simulink model "fsm_12B_with_contracts_PP"  (R2017b)
settings: Solver=FixedStepDiscrete  StartTime=0.0  StopTime=10  FixedStep=0.200000  RelTol=1e-3  EnableMultiTasking=on
model workspace (MAT data in the model file):
  MCOS : class17 (value not decoded)
  already_pp = 1
  compositionalMap : struct (value not decoded)
  MCOS : class17 (value not decoded)
  MCOS : class17 (value not decoded)
  verificationResults : struct (value not decoded)
undefined symbols (not defined in the file): contractAfterSimulation, contractBeforeSimulation, ContractBlock, ContractGuaranteeBlock, ContractValidatorBlock, saveValidatorParameters
(part 2 of 2)

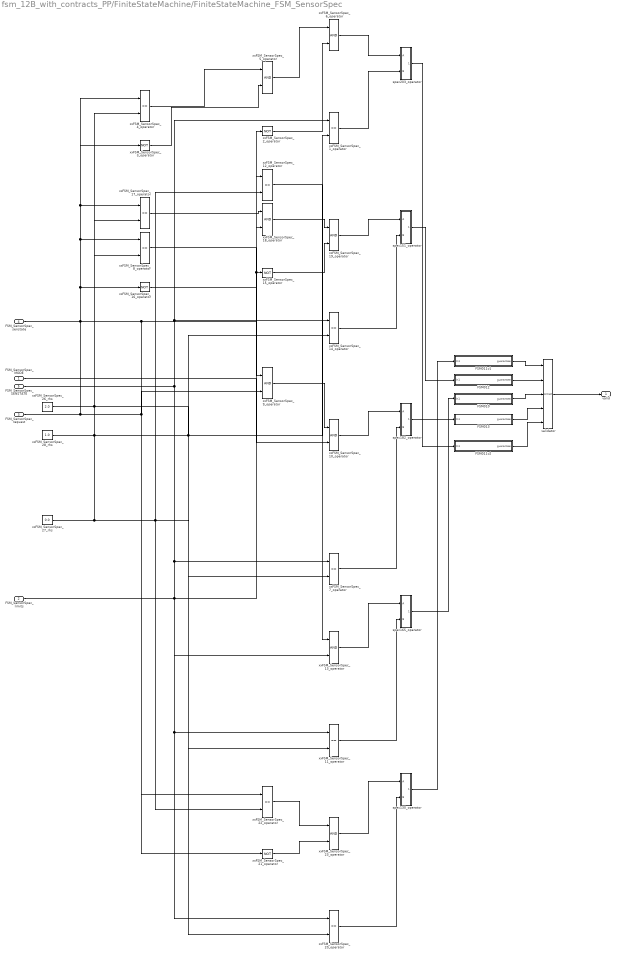
== system fsm_12B_with_contracts_PP/FiniteStateMachine/FiniteStateMachine_FSM_SensorSpec ==
  FSM_SensorSpec_MODE : Inport  OutDataTypeStr=boolean
  FSM_SensorSpec_limits : Inport  Port=2  OutDataTypeStr=boolean
  FSM_SensorSpec_request : Inport  Port=3  OutDataTypeStr=boolean
  FSM_SensorSpec_senstate : Inport  Port=4  OutDataTypeStr=double
  FSM_SensorSpec_SENSTATE : Inport  Port=5  OutDataTypeStr=double
  FSM010 : Subsystem  TreatAsAtomicUnit=on  mask(ContractGuaranteeBlock){ContractBlockType=ContractGuaranteeBlock}
      mask init:
      | set_param(gcb, 'LinkStatus', 'none');
      mask DialogControl DescTextVar Prompt: Guarantee block
  FSM011v1 : Subsystem  TreatAsAtomicUnit=on  mask(ContractGuaranteeBlock){ContractBlockType=ContractGuaranteeBlock}
      mask init:
      | set_param(gcb, 'LinkStatus', 'none');
      mask DialogControl DescTextVar Prompt: Guarantee block
      mask DialogControl Display_counter_example_as_signals Prompt: Display counter example as signals
      mask DialogControl Display_counter_example_as_signals Callback: displayCexSignals(1, 1);
      mask DialogControl Display_counter_example_as_tables Prompt: Display counter example as tables
      mask DialogControl Display_counter_example_as_tables Callback: displayCexTables(1, 1);
      mask DialogControl Display_counter_example_as_HTML_tables Prompt: Display counter example as HTML tables
      mask DialogControl Display_counter_example_as_HTML_tables Callback: displayCexHtmlTables(1, 1);
      mask DialogControl Generate_an_outer_model_for_the_counter_example Prompt: Generate an outer model for the counter example
      mask DialogControl Generate_an_outer_model_for_the_counter_example Callback: generateModelWithSignalBuilders(1, 1, 2);
      mask DialogControl Generate_an_inner_model_for_the_counter_example Prompt: Generate an inner model for the counter example
      mask DialogControl Generate_an_inner_model_for_the_counter_example Callback: generateModelWithSignalBuilders(1, 1, 1);
  FSM011v2 : Subsystem  TreatAsAtomicUnit=on  mask(ContractGuaranteeBlock){ContractBlockType=ContractGuaranteeBlock}
      mask init:
      | set_param(gcb, 'LinkStatus', 'none');
      mask DialogControl DescTextVar Prompt: Guarantee block
  FSM012 : Subsystem  TreatAsAtomicUnit=on  mask(ContractGuaranteeBlock){ContractBlockType=ContractGuaranteeBlock}
      mask init:
      | set_param(gcb, 'LinkStatus', 'none');
      mask DialogControl DescTextVar Prompt: Guarantee block
  FSM013 : Subsystem  TreatAsAtomicUnit=on  mask(ContractGuaranteeBlock){ContractBlockType=ContractGuaranteeBlock}
      mask init:
      | set_param(gcb, 'LinkStatus', 'none');
      mask DialogControl DescTextVar Prompt: Guarantee block
  spec130_operator : Subsystem  TreatAsAtomicUnit=on
  spec151_operator : Subsystem  TreatAsAtomicUnit=on
  spec165_operator : Subsystem  TreatAsAtomicUnit=on
  spec182_operator : Subsystem  TreatAsAtomicUnit=on
  spec203_operator : Subsystem  TreatAsAtomicUnit=on
  validator : M-S-Function  LoadFcn=saveValidatorParameters(gcb);  InitFcn=contractBeforeSimulation();  StopFcn=contractAfterSimulation();  FunctionName=contract  mask(ContractValidatorBlock){assumePorts=0, guaranteePorts=5, modePorts=0, ContractBlockType=ContractValidatorBlock, createInportsCheckbox=off}
      mask prompts: assumePorts "Assume ports     :"; guaranteePorts "Guarantee ports :"; modePorts "Mode ports        :"; createInportsCheckbox "Create inports and connect them automatically"
      mask init:
      | set_param(gcb,'LinkStatus','none');
      | contract_callback('inputs_callback',gcb);
      mask DialogControl DescTextVar Prompt: The validator block implements the following logic: <br> <br> <b>Sofar</b>(assume<sub>1</sub> <b>&#8743;</b> assume<sub>2</sub> <b>&#8743;</b> ... assume<sub>k</sub>) <b>&rarr;</b> (guarantee<sub>1</sub> <b>&#8743;</b> guarantee<sub>2</sub> <b>&#8743;</b> ... guarantee<sub>m</sub> <b>&#8743;</b>  mode<sub>1</sub> <b>&#8743;</b> mode<sub>2</sub> <b>&#8743;</b> ... <b>&#8743;</b> mode<sub>n</sub> )<br> where mode<sub>i</sub> = require<sub>i</sub> <b>&rarr;</b> ensure<sub>i</sub>
      mask Display:
      | color('black');
      | port_label('input',1,'guarantee');
      | port_label('input',2,'guarantee');
      | port_label('input',3,'guarantee');
      | port_label('input',4,'guarantee');
      | port_label('input',5,'guarantee');
      | port_label('output',1,'valid');
  xxFSM_SensorSpec_10_operator : Logic  AllPortsSameDT=off  OutDataTypeStr=boolean
  xxFSM_SensorSpec_11_operator : RelationalOperator  Operator===  OutDataTypeStr=boolean  RndMeth=Simplest
  xxFSM_SensorSpec_12_operator : RelationalOperator  Operator===  OutDataTypeStr=boolean  RndMeth=Simplest
  xxFSM_SensorSpec_13_operator : Logic  AllPortsSameDT=off  OutDataTypeStr=boolean
  xxFSM_SensorSpec_14_operator : RelationalOperator  Operator===  OutDataTypeStr=boolean  RndMeth=Simplest
  xxFSM_SensorSpec_15_operator : Logic  Operator=NOT  AllPortsSameDT=off  OutDataTypeStr=boolean
  xxFSM_SensorSpec_16_operator : Logic  Operator=NOT  AllPortsSameDT=off  OutDataTypeStr=boolean
  xxFSM_SensorSpec_17_operator : RelationalOperator  Operator===  OutDataTypeStr=boolean  RndMeth=Simplest
  xxFSM_SensorSpec_18_operator : Logic  AllPortsSameDT=off  OutDataTypeStr=boolean
  xxFSM_SensorSpec_19_operator : Logic  AllPortsSameDT=off  OutDataTypeStr=boolean
  xxFSM_SensorSpec_1_operator : RelationalOperator  Operator===  OutDataTypeStr=boolean  RndMeth=Simplest
  xxFSM_SensorSpec_20_operator : RelationalOperator  Operator===  OutDataTypeStr=boolean  RndMeth=Simplest
  xxFSM_SensorSpec_21_operator : Logic  Operator=NOT  AllPortsSameDT=off  OutDataTypeStr=boolean
  xxFSM_SensorSpec_22_operator : RelationalOperator  Operator===  OutDataTypeStr=boolean  RndMeth=Simplest
  xxFSM_SensorSpec_23_operator : Logic  AllPortsSameDT=off  OutDataTypeStr=boolean
  xxFSM_SensorSpec_26_rhs : Constant  Value=2.0  OutDataTypeStr=double
  xxFSM_SensorSpec_27_rhs : Constant  Value=0.0  OutDataTypeStr=double
  xxFSM_SensorSpec_28_rhs : Constant  Value=1.0  OutDataTypeStr=double
  xxFSM_SensorSpec_2_operator : Logic  Operator=NOT  AllPortsSameDT=off  OutDataTypeStr=boolean
  xxFSM_SensorSpec_3_operator : Logic  Operator=NOT  AllPortsSameDT=off  OutDataTypeStr=boolean
  xxFSM_SensorSpec_4_operator : RelationalOperator  Operator===  OutDataTypeStr=boolean  RndMeth=Simplest
  xxFSM_SensorSpec_5_operator : Logic  AllPortsSameDT=off  OutDataTypeStr=boolean
  xxFSM_SensorSpec_6_operator : Logic  AllPortsSameDT=off  OutDataTypeStr=boolean
  xxFSM_SensorSpec_7_operator : RelationalOperator  Operator===  OutDataTypeStr=boolean  RndMeth=Simplest
  xxFSM_SensorSpec_8_operator : RelationalOperator  Operator===  OutDataTypeStr=boolean  RndMeth=Simplest
  xxFSM_SensorSpec_9_operator : Logic  AllPortsSameDT=off  OutDataTypeStr=boolean
  valid : Outport
  wires:
  validator/1 -> valid/1
  xxFSM_SensorSpec_8_operator/1 -> xxFSM_SensorSpec_9_operator/1
  xxFSM_SensorSpec_2_operator/1 -> xxFSM_SensorSpec_6_operator/2
  xxFSM_SensorSpec_5_operator/1 -> xxFSM_SensorSpec_6_operator/1
  xxFSM_SensorSpec_3_operator/1 -> xxFSM_SensorSpec_5_operator/2
  xxFSM_SensorSpec_4_operator/1 -> xxFSM_SensorSpec_5_operator/1
  xxFSM_SensorSpec_21_operator/1 -> xxFSM_SensorSpec_23_operator/2
  xxFSM_SensorSpec_22_operator/1 -> xxFSM_SensorSpec_23_operator/1
  xxFSM_SensorSpec_15_operator/1 -> xxFSM_SensorSpec_19_operator/2
  xxFSM_SensorSpec_18_operator/1 -> xxFSM_SensorSpec_19_operator/1
  xxFSM_SensorSpec_16_operator/1 -> xxFSM_SensorSpec_18_operator/2
  xxFSM_SensorSpec_17_operator/1 -> xxFSM_SensorSpec_18_operator/1
  xxFSM_SensorSpec_12_operator/1 -> xxFSM_SensorSpec_13_operator/1
  FSM_SensorSpec_MODE/1 -> xxFSM_SensorSpec_10_operator/2
  xxFSM_SensorSpec_9_operator/1 -> xxFSM_SensorSpec_10_operator/1
  FSM011v2/1(guarantee) -> validator/5
  FSM013/1(guarantee) -> validator/4
  FSM010/1(guarantee) -> validator/3
  FSM012/1(guarantee) -> validator/2
  FSM011v1/1(guarantee) -> validator/1
  xxFSM_SensorSpec_1_operator/1 -> spec203_operator/2(B)
  xxFSM_SensorSpec_6_operator/1 -> spec203_operator/1(A)
  xxFSM_SensorSpec_7_operator/1 -> spec182_operator/2(B)
  xxFSM_SensorSpec_10_operator/1 -> spec182_operator/1(A)
  xxFSM_SensorSpec_11_operator/1 -> spec165_operator/2(B)
  xxFSM_SensorSpec_13_operator/1 -> spec165_operator/1(A)
  xxFSM_SensorSpec_14_operator/1 -> spec151_operator/2(B)
  xxFSM_SensorSpec_19_operator/1 -> spec151_operator/1(A)
  xxFSM_SensorSpec_20_operator/1 -> spec130_operator/2(B)
  xxFSM_SensorSpec_23_operator/1 -> spec130_operator/1(A)
  spec203_operator/1(A_equal__equal__gt_B) -> FSM011v2/1(In1)
  spec182_operator/1(A_equal__equal__gt_B) -> FSM013/1(In1)
  spec165_operator/1(A_equal__equal__gt_B) -> FSM010/1(In1)
  spec151_operator/1(A_equal__equal__gt_B) -> FSM012/1(In1)
  spec130_operator/1(A_equal__equal__gt_B) -> FSM011v1/1(In1)
  xxFSM_SensorSpec_28_rhs/1 -> xxFSM_SensorSpec_20_operator/2, xxFSM_SensorSpec_1_operator/2, xxFSM_SensorSpec_14_operator/2, xxFSM_SensorSpec_8_operator/2
  FSM_SensorSpec_request/1 -> xxFSM_SensorSpec_9_operator/2, xxFSM_SensorSpec_21_operator/1, xxFSM_SensorSpec_3_operator/1, xxFSM_SensorSpec_16_operator/1
  xxFSM_SensorSpec_26_rhs/1 -> xxFSM_SensorSpec_17_operator/2, xxFSM_SensorSpec_11_operator/2
  FSM_SensorSpec_SENSTATE/1 -> xxFSM_SensorSpec_20_operator/1, xxFSM_SensorSpec_11_operator/1, xxFSM_SensorSpec_7_operator/1, xxFSM_SensorSpec_1_operator/1, xxFSM_SensorSpec_14_operator/1
  FSM_SensorSpec_limits/1 -> xxFSM_SensorSpec_2_operator/1, xxFSM_SensorSpec_15_operator/1, xxFSM_SensorSpec_13_operator/2
  xxFSM_SensorSpec_27_rhs/1 -> xxFSM_SensorSpec_7_operator/2, xxFSM_SensorSpec_22_operator/2, xxFSM_SensorSpec_12_operator/2, xxFSM_SensorSpec_4_operator/2
  FSM_SensorSpec_senstate/1 -> xxFSM_SensorSpec_22_operator/1, xxFSM_SensorSpec_12_operator/1, xxFSM_SensorSpec_4_operator/1, xxFSM_SensorSpec_17_operator/1, xxFSM_SensorSpec_8_operator/1

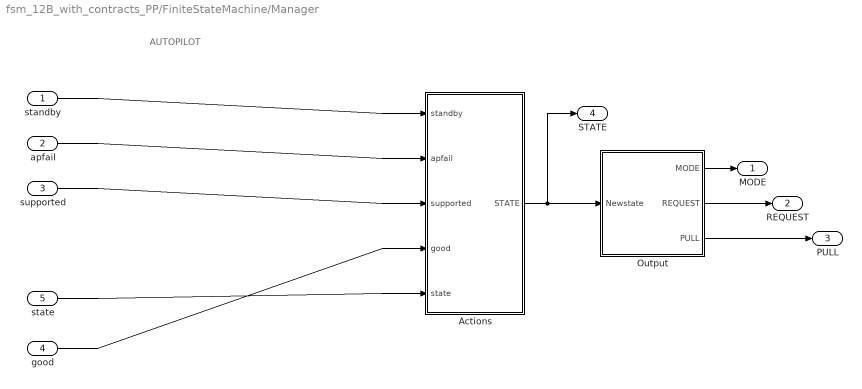
== system fsm_12B_with_contracts_PP/FiniteStateMachine/Manager ==
  note: AUTOPILOT
  standby : Inport
  apfail : Inport  Port=2
  supported : Inport  Port=3
  good : Inport  Port=4
  state : Inport  Port=5
  Actions : Subsystem  TreatAsAtomicUnit=on
  Output : Subsystem  TreatAsAtomicUnit=on
  MODE : Outport  VectorParamsAs1DForOutWhenUnconnected=off
  REQUEST : Outport  Port=2  VectorParamsAs1DForOutWhenUnconnected=off
  PULL : Outport  Port=3  VectorParamsAs1DForOutWhenUnconnected=off
  STATE : Outport  Port=4  VectorParamsAs1DForOutWhenUnconnected=off
  wires:
  Actions/1(STATE) -> STATE/1, Output/1(Newstate)
  apfail/1 -> Actions/2(apfail)
  state/1 -> Actions/5(state)
  supported/1 -> Actions/3(supported)
  good/1 -> Actions/4(good)
  standby/1 -> Actions/1(standby)
  Output/1(MODE) -> MODE/1
  Output/2(REQUEST) -> REQUEST/1
  Output/3(PULL) -> PULL/1

== system fsm_12B_with_contracts_PP/FiniteStateMachine/Sen ==
  note: SENSOR
  mode : Inport
  request : Inport  Port=2
  limits : Inport  Port=3
  senstate : Inport  Port=4
  Actions : Subsystem  TreatAsAtomicUnit=on
  Output : Subsystem  TreatAsAtomicUnit=on
  good : Outport  VectorParamsAs1DForOutWhenUnconnected=off
  SENSTATE : Outport  Port=2  VectorParamsAs1DForOutWhenUnconnected=off
  wires:
  Output/1(Good) -> good/1
  request/1 -> Actions/2(request)
  mode/1 -> Actions/1(mode)
  Actions/1(SENSTATE) -> Output/1(Newstate), SENSTATE/1
  senstate/1 -> Actions/4(senstate)
  limits/1 -> Actions/3(limits)

== system fsm_12B_with_contracts_PP/fsm_12B_FSMSpec/FSM001v1 ==
  In1 : Inport
  guarantee : Outport  OutDataTypeStr=boolean
  wires:
  In1/1 -> guarantee/1

== system fsm_12B_with_contracts_PP/fsm_12B_FSMSpec/FSM001v2 ==
  In1 : Inport
  guarantee : Outport  OutDataTypeStr=boolean
  wires:
  In1/1 -> guarantee/1

== system fsm_12B_with_contracts_PP/fsm_12B_FSMSpec/FSM001v3 ==
  In1 : Inport
  guarantee : Outport  OutDataTypeStr=boolean
  wires:
  In1/1 -> guarantee/1

== system fsm_12B_with_contracts_PP/fsm_12B_FSMSpec/HT_call ==
  HT_L : Inport
  HT_R : Inport  Port=2
  HT_X : Inport  Port=3  OutDataTypeStr=boolean
  OT_call : Subsystem  TreatAsAtomicUnit=on
  Y_operator : Logic  Operator=NOT  AllPortsSameDT=off  OutDataTypeStr=boolean
  xxHT_1_operator : Logic  Operator=NOT  AllPortsSameDT=off  OutDataTypeStr=boolean
  HT_Y : Outport
  wires:
  Y_operator/1 -> HT_Y/1
  HT_X/1 -> xxHT_1_operator/1
  OT_call/1(OT_Y) -> Y_operator/1
  xxHT_1_operator/1 -> OT_call/3(OT_X)
  HT_R/1 -> OT_call/2(OT_R)
  HT_L/1 -> OT_call/1(OT_L)

== system fsm_12B_with_contracts_PP/fsm_12B_FSMSpec/HT_call1 ==
  HT_L : Inport
  HT_R : Inport  Port=2
  HT_X : Inport  Port=3  OutDataTypeStr=boolean
  OT_call : Subsystem  TreatAsAtomicUnit=on
  Y_operator : Logic  Operator=NOT  AllPortsSameDT=off  OutDataTypeStr=boolean
  xxHT_1_operator : Logic  Operator=NOT  AllPortsSameDT=off  OutDataTypeStr=boolean
  HT_Y : Outport
  wires:
  Y_operator/1 -> HT_Y/1
  HT_X/1 -> xxHT_1_operator/1
  OT_call/1(OT_Y) -> Y_operator/1
  xxHT_1_operator/1 -> OT_call/3(OT_X)
  HT_R/1 -> OT_call/2(OT_R)
  HT_L/1 -> OT_call/1(OT_L)

== system fsm_12B_with_contracts_PP/fsm_12B_FSMSpec/spec166_operator ==
  A : Inport
  B : Inport  Port=2
  Logical_newline_Operator : Logic  Operator=OR  AllPortsSameDT=off  OutDataTypeStr=boolean
  Logical_newline_Operator1 : Logic  Operator=NOT  AllPortsSameDT=off  OutDataTypeStr=boolean
  A_equal__equal__gt_B : Outport  VectorParamsAs1DForOutWhenUnconnected=off
  wires:
  B/1 -> Logical_newline_Operator/2
  A/1 -> Logical_newline_Operator1/1
  Logical_newline_Operator/1 -> A_equal__equal__gt_B/1
  Logical_newline_Operator1/1 -> Logical_newline_Operator/1

== system fsm_12B_with_contracts_PP/fsm_12B_FSMSpec/spec194_operator ==
  A : Inport
  B : Inport  Port=2
  Logical_newline_Operator : Logic  Operator=OR  AllPortsSameDT=off  OutDataTypeStr=boolean
  Logical_newline_Operator1 : Logic  Operator=NOT  AllPortsSameDT=off  OutDataTypeStr=boolean
  A_equal__equal__gt_B : Outport  VectorParamsAs1DForOutWhenUnconnected=off
  wires:
  B/1 -> Logical_newline_Operator/2
  A/1 -> Logical_newline_Operator1/1
  Logical_newline_Operator/1 -> A_equal__equal__gt_B/1
  Logical_newline_Operator1/1 -> Logical_newline_Operator/1

== system fsm_12B_with_contracts_PP/fsm_12B_FSMSpec/spec222_operator ==
  A : Inport
  B : Inport  Port=2
  Logical_newline_Operator : Logic  Operator=OR  AllPortsSameDT=off  OutDataTypeStr=boolean
  Logical_newline_Operator1 : Logic  Operator=NOT  AllPortsSameDT=off  OutDataTypeStr=boolean
  A_equal__equal__gt_B : Outport  VectorParamsAs1DForOutWhenUnconnected=off
  wires:
  B/1 -> Logical_newline_Operator/2
  A/1 -> Logical_newline_Operator1/1
  Logical_newline_Operator/1 -> A_equal__equal__gt_B/1
  Logical_newline_Operator1/1 -> Logical_newline_Operator/1

== system fsm_12B_with_contracts_PP/FiniteStateMachine/FiniteStateMachine_FSM_AutopilotSpec1/FSM002 ==
  In1 : Inport
  guarantee : Outport  OutDataTypeStr=boolean
  wires:
  In1/1 -> guarantee/1

== system fsm_12B_with_contracts_PP/FiniteStateMachine/FiniteStateMachine_FSM_AutopilotSpec1/FSM003 ==
  In1 : Inport
  guarantee : Outport  OutDataTypeStr=boolean
  wires:
  In1/1 -> guarantee/1

== system fsm_12B_with_contracts_PP/FiniteStateMachine/FiniteStateMachine_FSM_AutopilotSpec1/FSM003v2 ==
  In1 : Inport
  guarantee : Outport  OutDataTypeStr=boolean
  wires:
  In1/1 -> guarantee/1

== system fsm_12B_with_contracts_PP/FiniteStateMachine/FiniteStateMachine_FSM_AutopilotSpec1/FSM004 ==
  In1 : Inport
  guarantee : Outport  OutDataTypeStr=boolean
  wires:
  In1/1 -> guarantee/1

== system fsm_12B_with_contracts_PP/FiniteStateMachine/FiniteStateMachine_FSM_AutopilotSpec1/FSM004v2 ==
  In1 : Inport
  guarantee : Outport  OutDataTypeStr=boolean
  wires:
  In1/1 -> guarantee/1

== system fsm_12B_with_contracts_PP/FiniteStateMachine/FiniteStateMachine_FSM_AutopilotSpec1/FSM005 ==
  In1 : Inport
  guarantee : Outport  OutDataTypeStr=boolean
  wires:
  In1/1 -> guarantee/1

== system fsm_12B_with_contracts_PP/FiniteStateMachine/FiniteStateMachine_FSM_AutopilotSpec1/FSM006 ==
  In1 : Inport
  guarantee : Outport  OutDataTypeStr=boolean
  wires:
  In1/1 -> guarantee/1

== system fsm_12B_with_contracts_PP/FiniteStateMachine/FiniteStateMachine_FSM_AutopilotSpec1/FSM007 ==
  In1 : Inport
  guarantee : Outport  OutDataTypeStr=boolean
  wires:
  In1/1 -> guarantee/1

== system fsm_12B_with_contracts_PP/FiniteStateMachine/FiniteStateMachine_FSM_AutopilotSpec1/FSM007v2 ==
  In1 : Inport
  guarantee : Outport  OutDataTypeStr=boolean
  wires:
  In1/1 -> guarantee/1

== system fsm_12B_with_contracts_PP/FiniteStateMachine/FiniteStateMachine_FSM_AutopilotSpec1/FSM008v1 ==
  In1 : Inport
  guarantee : Outport  OutDataTypeStr=boolean
  wires:
  In1/1 -> guarantee/1

== system fsm_12B_with_contracts_PP/FiniteStateMachine/FiniteStateMachine_FSM_AutopilotSpec1/FSM008v2 ==
  In1 : Inport
  guarantee : Outport  OutDataTypeStr=boolean
  wires:
  In1/1 -> guarantee/1

== system fsm_12B_with_contracts_PP/FiniteStateMachine/FiniteStateMachine_FSM_AutopilotSpec1/FSM009 ==
  In1 : Inport
  guarantee : Outport  OutDataTypeStr=boolean
  wires:
  In1/1 -> guarantee/1

== system fsm_12B_with_contracts_PP/FiniteStateMachine/FiniteStateMachine_FSM_AutopilotSpec1/spec129_operator ==
  A : Inport
  B : Inport  Port=2
  Logical_newline_Operator : Logic  Operator=OR  AllPortsSameDT=off  OutDataTypeStr=boolean
  Logical_newline_Operator1 : Logic  Operator=NOT  AllPortsSameDT=off  OutDataTypeStr=boolean
  A_equal__equal__gt_B : Outport  VectorParamsAs1DForOutWhenUnconnected=off
  wires:
  Logical_newline_Operator1/1 -> Logical_newline_Operator/1
  Logical_newline_Operator/1 -> A_equal__equal__gt_B/1
  A/1 -> Logical_newline_Operator1/1
  B/1 -> Logical_newline_Operator/2

== system fsm_12B_with_contracts_PP/FiniteStateMachine/FiniteStateMachine_FSM_AutopilotSpec1/spec143_operator ==
  A : Inport
  B : Inport  Port=2
  Logical_newline_Operator : Logic  Operator=OR  AllPortsSameDT=off  OutDataTypeStr=boolean
  Logical_newline_Operator1 : Logic  Operator=NOT  AllPortsSameDT=off  OutDataTypeStr=boolean
  A_equal__equal__gt_B : Outport  VectorParamsAs1DForOutWhenUnconnected=off
  wires:
  Logical_newline_Operator1/1 -> Logical_newline_Operator/1
  Logical_newline_Operator/1 -> A_equal__equal__gt_B/1
  A/1 -> Logical_newline_Operator1/1
  B/1 -> Logical_newline_Operator/2

== system fsm_12B_with_contracts_PP/FiniteStateMachine/FiniteStateMachine_FSM_AutopilotSpec1/spec160_operator ==
  A : Inport
  B : Inport  Port=2
  Logical_newline_Operator : Logic  Operator=OR  AllPortsSameDT=off  OutDataTypeStr=boolean
  Logical_newline_Operator1 : Logic  Operator=NOT  AllPortsSameDT=off  OutDataTypeStr=boolean
  A_equal__equal__gt_B : Outport  VectorParamsAs1DForOutWhenUnconnected=off
  wires:
  Logical_newline_Operator1/1 -> Logical_newline_Operator/1
  Logical_newline_Operator/1 -> A_equal__equal__gt_B/1
  A/1 -> Logical_newline_Operator1/1
  B/1 -> Logical_newline_Operator/2

== system fsm_12B_with_contracts_PP/FiniteStateMachine/FiniteStateMachine_FSM_AutopilotSpec1/spec182_operator ==
  A : Inport
  B : Inport  Port=2
  Logical_newline_Operator : Logic  Operator=OR  AllPortsSameDT=off  OutDataTypeStr=boolean
  Logical_newline_Operator1 : Logic  Operator=NOT  AllPortsSameDT=off  OutDataTypeStr=boolean
  A_equal__equal__gt_B : Outport  VectorParamsAs1DForOutWhenUnconnected=off
  wires:
  Logical_newline_Operator1/1 -> Logical_newline_Operator/1
  Logical_newline_Operator/1 -> A_equal__equal__gt_B/1
  A/1 -> Logical_newline_Operator1/1
  B/1 -> Logical_newline_Operator/2

== system fsm_12B_with_contracts_PP/FiniteStateMachine/FiniteStateMachine_FSM_AutopilotSpec1/spec198_operator ==
  A : Inport
  B : Inport  Port=2
  Logical_newline_Operator : Logic  Operator=OR  AllPortsSameDT=off  OutDataTypeStr=boolean
  Logical_newline_Operator1 : Logic  Operator=NOT  AllPortsSameDT=off  OutDataTypeStr=boolean
  A_equal__equal__gt_B : Outport  VectorParamsAs1DForOutWhenUnconnected=off
  wires:
  Logical_newline_Operator1/1 -> Logical_newline_Operator/1
  Logical_newline_Operator/1 -> A_equal__equal__gt_B/1
  A/1 -> Logical_newline_Operator1/1
  B/1 -> Logical_newline_Operator/2

== system fsm_12B_with_contracts_PP/FiniteStateMachine/FiniteStateMachine_FSM_AutopilotSpec1/spec212_operator ==
  A : Inport
  B : Inport  Port=2
  Logical_newline_Operator : Logic  Operator=OR  AllPortsSameDT=off  OutDataTypeStr=boolean
  Logical_newline_Operator1 : Logic  Operator=NOT  AllPortsSameDT=off  OutDataTypeStr=boolean
  A_equal__equal__gt_B : Outport  VectorParamsAs1DForOutWhenUnconnected=off
  wires:
  Logical_newline_Operator1/1 -> Logical_newline_Operator/1
  Logical_newline_Operator/1 -> A_equal__equal__gt_B/1
  A/1 -> Logical_newline_Operator1/1
  B/1 -> Logical_newline_Operator/2

== system fsm_12B_with_contracts_PP/FiniteStateMachine/FiniteStateMachine_FSM_AutopilotSpec1/spec233_operator ==
  A : Inport
  B : Inport  Port=2
  Logical_newline_Operator : Logic  Operator=OR  AllPortsSameDT=off  OutDataTypeStr=boolean
  Logical_newline_Operator1 : Logic  Operator=NOT  AllPortsSameDT=off  OutDataTypeStr=boolean
  A_equal__equal__gt_B : Outport  VectorParamsAs1DForOutWhenUnconnected=off
  wires:
  Logical_newline_Operator1/1 -> Logical_newline_Operator/1
  Logical_newline_Operator/1 -> A_equal__equal__gt_B/1
  A/1 -> Logical_newline_Operator1/1
  B/1 -> Logical_newline_Operator/2

== system fsm_12B_with_contracts_PP/FiniteStateMachine/FiniteStateMachine_FSM_AutopilotSpec1/spec254_operator ==
  A : Inport
  B : Inport  Port=2
  Logical_newline_Operator : Logic  Operator=OR  AllPortsSameDT=off  OutDataTypeStr=boolean
  Logical_newline_Operator1 : Logic  Operator=NOT  AllPortsSameDT=off  OutDataTypeStr=boolean
  A_equal__equal__gt_B : Outport  VectorParamsAs1DForOutWhenUnconnected=off
  wires:
  Logical_newline_Operator1/1 -> Logical_newline_Operator/1
  Logical_newline_Operator/1 -> A_equal__equal__gt_B/1
  A/1 -> Logical_newline_Operator1/1
  B/1 -> Logical_newline_Operator/2

== system fsm_12B_with_contracts_PP/FiniteStateMachine/FiniteStateMachine_FSM_AutopilotSpec1/spec271_operator ==
  A : Inport
  B : Inport  Port=2
  Logical_newline_Operator : Logic  Operator=OR  AllPortsSameDT=off  OutDataTypeStr=boolean
  Logical_newline_Operator1 : Logic  Operator=NOT  AllPortsSameDT=off  OutDataTypeStr=boolean
  A_equal__equal__gt_B : Outport  VectorParamsAs1DForOutWhenUnconnected=off
  wires:
  Logical_newline_Operator1/1 -> Logical_newline_Operator/1
  Logical_newline_Operator/1 -> A_equal__equal__gt_B/1
  A/1 -> Logical_newline_Operator1/1
  B/1 -> Logical_newline_Operator/2

== system fsm_12B_with_contracts_PP/FiniteStateMachine/FiniteStateMachine_FSM_AutopilotSpec1/spec287_operator ==
  A : Inport
  B : Inport  Port=2
  Logical_newline_Operator : Logic  Operator=OR  AllPortsSameDT=off  OutDataTypeStr=boolean
  Logical_newline_Operator1 : Logic  Operator=NOT  AllPortsSameDT=off  OutDataTypeStr=boolean
  A_equal__equal__gt_B : Outport  VectorParamsAs1DForOutWhenUnconnected=off
  wires:
  Logical_newline_Operator1/1 -> Logical_newline_Operator/1
  Logical_newline_Operator/1 -> A_equal__equal__gt_B/1
  A/1 -> Logical_newline_Operator1/1
  B/1 -> Logical_newline_Operator/2

== system fsm_12B_with_contracts_PP/FiniteStateMachine/FiniteStateMachine_FSM_AutopilotSpec1/spec309_operator ==
  A : Inport
  B : Inport  Port=2
  Logical_newline_Operator : Logic  Operator=OR  AllPortsSameDT=off  OutDataTypeStr=boolean
  Logical_newline_Operator1 : Logic  Operator=NOT  AllPortsSameDT=off  OutDataTypeStr=boolean
  A_equal__equal__gt_B : Outport  VectorParamsAs1DForOutWhenUnconnected=off
  wires:
  Logical_newline_Operator1/1 -> Logical_newline_Operator/1
  Logical_newline_Operator/1 -> A_equal__equal__gt_B/1
  A/1 -> Logical_newline_Operator1/1
  B/1 -> Logical_newline_Operator/2

== system fsm_12B_with_contracts_PP/FiniteStateMachine/FiniteStateMachine_FSM_AutopilotSpec1/spec326_operator ==
  A : Inport
  B : Inport  Port=2
  Logical_newline_Operator : Logic  Operator=OR  AllPortsSameDT=off  OutDataTypeStr=boolean
  Logical_newline_Operator1 : Logic  Operator=NOT  AllPortsSameDT=off  OutDataTypeStr=boolean
  A_equal__equal__gt_B : Outport  VectorParamsAs1DForOutWhenUnconnected=off
  wires:
  Logical_newline_Operator1/1 -> Logical_newline_Operator/1
  Logical_newline_Operator/1 -> A_equal__equal__gt_B/1
  A/1 -> Logical_newline_Operator1/1
  B/1 -> Logical_newline_Operator/2

== system fsm_12B_with_contracts_PP/FiniteStateMachine/FiniteStateMachine_FSM_SensorSpec/FSM010 ==
  In1 : Inport
  guarantee : Outport  OutDataTypeStr=boolean
  wires:
  In1/1 -> guarantee/1

== system fsm_12B_with_contracts_PP/FiniteStateMachine/FiniteStateMachine_FSM_SensorSpec/FSM011v1 ==
  In1 : Inport
  guarantee : Outport  OutDataTypeStr=boolean
  wires:
  In1/1 -> guarantee/1

== system fsm_12B_with_contracts_PP/FiniteStateMachine/FiniteStateMachine_FSM_SensorSpec/FSM011v2 ==
  In1 : Inport
  guarantee : Outport  OutDataTypeStr=boolean
  wires:
  In1/1 -> guarantee/1

== system fsm_12B_with_contracts_PP/FiniteStateMachine/FiniteStateMachine_FSM_SensorSpec/FSM012 ==
  In1 : Inport
  guarantee : Outport  OutDataTypeStr=boolean
  wires:
  In1/1 -> guarantee/1

== system fsm_12B_with_contracts_PP/FiniteStateMachine/FiniteStateMachine_FSM_SensorSpec/FSM013 ==
  In1 : Inport
  guarantee : Outport  OutDataTypeStr=boolean
  wires:
  In1/1 -> guarantee/1

== system fsm_12B_with_contracts_PP/FiniteStateMachine/FiniteStateMachine_FSM_SensorSpec/spec130_operator ==
  A : Inport
  B : Inport  Port=2
  Logical_newline_Operator : Logic  Operator=OR  AllPortsSameDT=off  OutDataTypeStr=boolean
  Logical_newline_Operator1 : Logic  Operator=NOT  AllPortsSameDT=off  OutDataTypeStr=boolean
  A_equal__equal__gt_B : Outport  VectorParamsAs1DForOutWhenUnconnected=off
  wires:
  B/1 -> Logical_newline_Operator/2
  A/1 -> Logical_newline_Operator1/1
  Logical_newline_Operator/1 -> A_equal__equal__gt_B/1
  Logical_newline_Operator1/1 -> Logical_newline_Operator/1

== system fsm_12B_with_contracts_PP/FiniteStateMachine/FiniteStateMachine_FSM_SensorSpec/spec151_operator ==
  A : Inport
  B : Inport  Port=2
  Logical_newline_Operator : Logic  Operator=OR  AllPortsSameDT=off  OutDataTypeStr=boolean
  Logical_newline_Operator1 : Logic  Operator=NOT  AllPortsSameDT=off  OutDataTypeStr=boolean
  A_equal__equal__gt_B : Outport  VectorParamsAs1DForOutWhenUnconnected=off
  wires:
  B/1 -> Logical_newline_Operator/2
  A/1 -> Logical_newline_Operator1/1
  Logical_newline_Operator/1 -> A_equal__equal__gt_B/1
  Logical_newline_Operator1/1 -> Logical_newline_Operator/1

== system fsm_12B_with_contracts_PP/FiniteStateMachine/FiniteStateMachine_FSM_SensorSpec/spec165_operator ==
  A : Inport
  B : Inport  Port=2
  Logical_newline_Operator : Logic  Operator=OR  AllPortsSameDT=off  OutDataTypeStr=boolean
  Logical_newline_Operator1 : Logic  Operator=NOT  AllPortsSameDT=off  OutDataTypeStr=boolean
  A_equal__equal__gt_B : Outport  VectorParamsAs1DForOutWhenUnconnected=off
  wires:
  B/1 -> Logical_newline_Operator/2
  A/1 -> Logical_newline_Operator1/1
  Logical_newline_Operator/1 -> A_equal__equal__gt_B/1
  Logical_newline_Operator1/1 -> Logical_newline_Operator/1

== system fsm_12B_with_contracts_PP/FiniteStateMachine/FiniteStateMachine_FSM_SensorSpec/spec182_operator ==
  A : Inport
  B : Inport  Port=2
  Logical_newline_Operator : Logic  Operator=OR  AllPortsSameDT=off  OutDataTypeStr=boolean
  Logical_newline_Operator1 : Logic  Operator=NOT  AllPortsSameDT=off  OutDataTypeStr=boolean
  A_equal__equal__gt_B : Outport  VectorParamsAs1DForOutWhenUnconnected=off
  wires:
  B/1 -> Logical_newline_Operator/2
  A/1 -> Logical_newline_Operator1/1
  Logical_newline_Operator/1 -> A_equal__equal__gt_B/1
  Logical_newline_Operator1/1 -> Logical_newline_Operator/1

== system fsm_12B_with_contracts_PP/FiniteStateMachine/FiniteStateMachine_FSM_SensorSpec/spec203_operator ==
  A : Inport
  B : Inport  Port=2
  Logical_newline_Operator : Logic  Operator=OR  AllPortsSameDT=off  OutDataTypeStr=boolean
  Logical_newline_Operator1 : Logic  Operator=NOT  AllPortsSameDT=off  OutDataTypeStr=boolean
  A_equal__equal__gt_B : Outport  VectorParamsAs1DForOutWhenUnconnected=off
  wires:
  B/1 -> Logical_newline_Operator/2
  A/1 -> Logical_newline_Operator1/1
  Logical_newline_Operator/1 -> A_equal__equal__gt_B/1
  Logical_newline_Operator1/1 -> Logical_newline_Operator/1

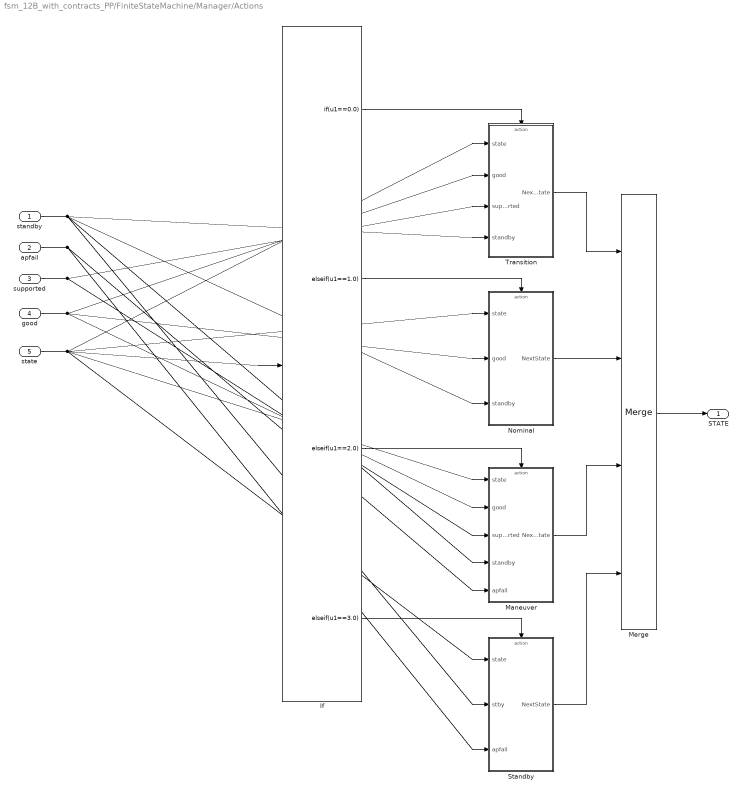
== system fsm_12B_with_contracts_PP/FiniteStateMachine/Manager/Actions ==
  standby : Inport
  apfail : Inport  Port=2
  supported : Inport  Port=3
  good : Inport  Port=4
  state : Inport  Port=5
  If : If  IfExpression=u1==0.0  ElseIfExpressions=u1==1.0, u1==2.0, u1==3.0  ShowElse=off
  Maneuver : Subsystem  TreatAsAtomicUnit=on
  Merge : Merge  Inputs=4
  Nominal : Subsystem  TreatAsAtomicUnit=on
  Standby : Subsystem  TreatAsAtomicUnit=on
  Transition : Subsystem  TreatAsAtomicUnit=on
  STATE : Outport  VectorParamsAs1DForOutWhenUnconnected=off
  wires:
  state/1 -> If/1, Transition/1(state), Nominal/1(state), Maneuver/1(state), Standby/1(state)
  Standby/1(NextState) -> Merge/4
  Maneuver/1(NextState) -> Merge/3
  Merge/1 -> STATE/1
  Transition/1(NextState) -> Merge/1
  Nominal/1(NextState) -> Merge/2
  If/2 -> Nominal/Action
  If/3 -> Maneuver/Action
  If/4 -> Standby/Action
  apfail/1 -> Maneuver/5(apfail), Standby/3(apfail)
  If/1 -> Transition/Action
  supported/1 -> Transition/3(supported), Maneuver/3(supported)
  good/1 -> Transition/2(good), Nominal/2(good), Maneuver/2(good)
  standby/1 -> Transition/4(standby), Nominal/3(standby), Maneuver/4(standby), Standby/2(stby)

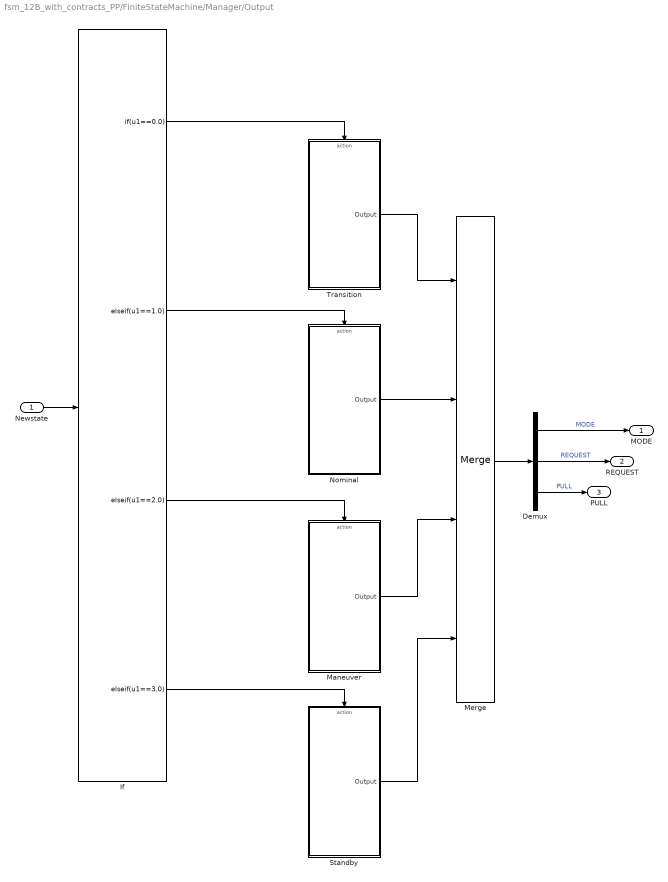
== system fsm_12B_with_contracts_PP/FiniteStateMachine/Manager/Output ==
  Newstate : Inport
  Demux : Demux  Outputs=3
  If : If  IfExpression=u1==0.0  ElseIfExpressions=u1==1.0, u1==2.0, u1==3.0  ShowElse=off
  Maneuver : Subsystem  TreatAsAtomicUnit=on
  Merge : Merge  Inputs=4
  Nominal : Subsystem  TreatAsAtomicUnit=on
  Standby : Subsystem  TreatAsAtomicUnit=on
  Transition : Subsystem  TreatAsAtomicUnit=on
  MODE : Outport  VectorParamsAs1DForOutWhenUnconnected=off
  REQUEST : Outport  Port=2  VectorParamsAs1DForOutWhenUnconnected=off
  PULL : Outport  Port=3  VectorParamsAs1DForOutWhenUnconnected=off
  wires:
  Demux/2 -> REQUEST/1  "REQUEST"
  Demux/1 -> MODE/1  "MODE"
  Demux/3 -> PULL/1  "PULL"
  Merge/1 -> Demux/1
  Nominal/1(Output) -> Merge/2
  Maneuver/1(Output) -> Merge/3
  If/2 -> Nominal/Action
  Transition/1(Output) -> Merge/1
  If/3 -> Maneuver/Action
  Standby/1(Output) -> Merge/4
  If/1 -> Transition/Action
  Newstate/1 -> If/1
  If/4 -> Standby/Action

== system fsm_12B_with_contracts_PP/FiniteStateMachine/Sen/Actions ==
  mode : Inport
  request : Inport  Port=2
  limits : Inport  Port=3
  senstate : Inport  Port=4
  Fault : Subsystem  TreatAsAtomicUnit=on
  If : If  IfExpression=u1==0.0  ElseIfExpressions=u1==1.0, u1==2.0  ShowElse=off
  Merge : Merge  Inputs=3
  Nominal : Subsystem  TreatAsAtomicUnit=on
  Transition : Subsystem  TreatAsAtomicUnit=on
  SENSTATE : Outport  VectorParamsAs1DForOutWhenUnconnected=off
  wires:
  senstate/1 -> If/1, Nominal/1(state), Transition/1(state), Fault/1(state)
  Fault/1(NextState) -> Merge/3
  Merge/1 -> SENSTATE/1
  Nominal/1(NextState) -> Merge/1
  Transition/1(NextState) -> Merge/2
  If/2 -> Transition/Action
  If/3 -> Fault/Action
  mode/1 -> Transition/3(mode)
  If/1 -> Nominal/Action
  request/1 -> Nominal/2(request), Transition/2(request), Fault/2(request)
  limits/1 -> Nominal/3(limits), Fault/3(limits)

== system fsm_12B_with_contracts_PP/FiniteStateMachine/Sen/Output ==
  Newstate : Inport
  Constant12 : Constant  OutDataTypeStr=boolean
  Constant6 : Constant  Value=2
  Constant9 : Constant  Value=0  OutDataTypeStr=boolean
  RelationalOperator5 : RelationalOperator  Operator===  OutDataTypeStr=boolean  RndMeth=Nearest
  Switch2 : Switch  Criteria=u2 ~= 0
  Good : Outport  VectorParamsAs1DForOutWhenUnconnected=off
  wires:
  Constant6/1 -> RelationalOperator5/2
  RelationalOperator5/1 -> Switch2/2
  Constant9/1 -> Switch2/1
  Constant12/1 -> Switch2/3
  Switch2/1 -> Good/1
  Newstate/1 -> RelationalOperator5/1

== system fsm_12B_with_contracts_PP/fsm_12B_FSMSpec/HT_call/OT_call ==
  OT_L : Inport
  OT_R : Inport  Port=2
  OT_X : Inport  Port=3  OutDataTypeStr=boolean
  OTlore_call : Subsystem  TreatAsAtomicUnit=on
  delay_call : Subsystem  TreatAsAtomicUnit=on
  xxOT_1_operator : Sum  Inputs=+-  OutDataTypeStr=int32
  OT_Y : Outport
  wires:
  OTlore_call/1(OTlore_Y) -> OT_Y/1
  OT_L/1 -> xxOT_1_operator/1
  OT_X/1 -> delay_call/1(delay_X)
  delay_call/1(delay_Y) -> OTlore_call/2(OTlore_X)
  xxOT_1_operator/1 -> OTlore_call/1(OTlore_N)
  OT_R/1 -> xxOT_1_operator/2, delay_call/2(delay_R)

== system fsm_12B_with_contracts_PP/fsm_12B_FSMSpec/HT_call1/OT_call ==
  OT_L : Inport
  OT_R : Inport  Port=2
  OT_X : Inport  Port=3  OutDataTypeStr=boolean
  OTlore_call : Subsystem  TreatAsAtomicUnit=on
  delay_call : Subsystem  TreatAsAtomicUnit=on
  xxOT_1_operator : Sum  Inputs=+-  OutDataTypeStr=int32
  OT_Y : Outport
  wires:
  OTlore_call/1(OTlore_Y) -> OT_Y/1
  OT_L/1 -> xxOT_1_operator/1
  OT_X/1 -> delay_call/1(delay_X)
  delay_call/1(delay_Y) -> OTlore_call/2(OTlore_X)
  xxOT_1_operator/1 -> OTlore_call/1(OTlore_N)
  OT_R/1 -> xxOT_1_operator/2, delay_call/2(delay_R)

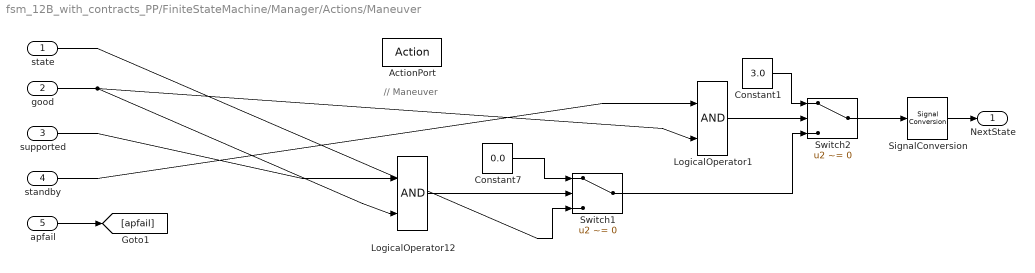
== system fsm_12B_with_contracts_PP/FiniteStateMachine/Manager/Actions/Maneuver ==
  note: // Maneuver
  state : Inport
  good : Inport  Port=2
  supported : Inport  Port=3
  standby : Inport  Port=4
  apfail : Inport  Port=5
  ActionPort : ActionPort
  Constant1 : Constant  Value=3.0
  Constant7 : Constant  Value=0.0
  LogicalOperator1 : Logic  IconShape=distinctive  AllPortsSameDT=off  OutDataTypeStr=boolean
  LogicalOperator12 : Logic  IconShape=distinctive  AllPortsSameDT=off  OutDataTypeStr=boolean
  SignalConversion : SignalConversion  OverrideOpt=off
  Switch1 : Switch  Criteria=u2 ~= 0
  Switch2 : Switch  Criteria=u2 ~= 0
  NextState : Outport  VectorParamsAs1DForOutWhenUnconnected=off
  wires:
  supported/1 -> LogicalOperator12/1
  LogicalOperator12/1 -> Switch1/2
  state/1 -> Switch1/3
  Constant7/1 -> Switch1/1
  LogicalOperator1/1 -> Switch2/2
  Constant1/1 -> Switch2/1
  Switch2/1 -> SignalConversion/1
  SignalConversion/1 -> NextState/1
  apfail/1 -> [apfail]
  good/1 -> LogicalOperator12/2, LogicalOperator1/2
  standby/1 -> LogicalOperator1/1
  Switch1/1 -> Switch2/3

== system fsm_12B_with_contracts_PP/FiniteStateMachine/Manager/Actions/Nominal ==
  note: // Nominal
  state : Inport
  good : Inport  Port=2
  standby : Inport  Port=3
  ActionPort : ActionPort
  Constant1 : Constant  Value=3.0
  Constant7 : Constant  Value=2.0
  LogicalOperator12 : Logic  Operator=NOT  IconShape=distinctive  AllPortsSameDT=off  OutDataTypeStr=boolean
  SignalConversion : SignalConversion  OverrideOpt=off
  Switch1 : Switch  Criteria=u2 ~= 0
  Switch2 : Switch  Criteria=u2 ~= 0
  NextState : Outport  VectorParamsAs1DForOutWhenUnconnected=off
  wires:
  SignalConversion/1 -> NextState/1
  Switch2/1 -> SignalConversion/1
  Switch1/1 -> Switch2/3
  Constant1/1 -> Switch2/1
  standby/1 -> Switch2/2
  Constant7/1 -> Switch1/1
  state/1 -> Switch1/3
  LogicalOperator12/1 -> Switch1/2
  good/1 -> LogicalOperator12/1

== system fsm_12B_with_contracts_PP/FiniteStateMachine/Manager/Actions/Standby ==
  note: // Standby
  state : Inport
  stby : Inport  Port=2
  apfail : Inport  Port=3
  ActionPort : ActionPort
  Constant1 : Constant  Value=2.0
  Constant7 : Constant  Value=0.0
  LogicalOperator12 : Logic  Operator=NOT  IconShape=distinctive  AllPortsSameDT=off  OutDataTypeStr=boolean
  SignalConversion : SignalConversion  OverrideOpt=off
  Switch1 : Switch  Criteria=u2 ~= 0
  Switch2 : Switch  Criteria=u2 ~= 0
  NextState : Outport  VectorParamsAs1DForOutWhenUnconnected=off
  wires:
  SignalConversion/1 -> NextState/1
  Switch2/1 -> SignalConversion/1
  Switch1/1 -> Switch2/3
  Constant1/1 -> Switch2/1
  apfail/1 -> Switch2/2
  Constant7/1 -> Switch1/1
  state/1 -> Switch1/3
  LogicalOperator12/1 -> Switch1/2
  stby/1 -> LogicalOperator12/1

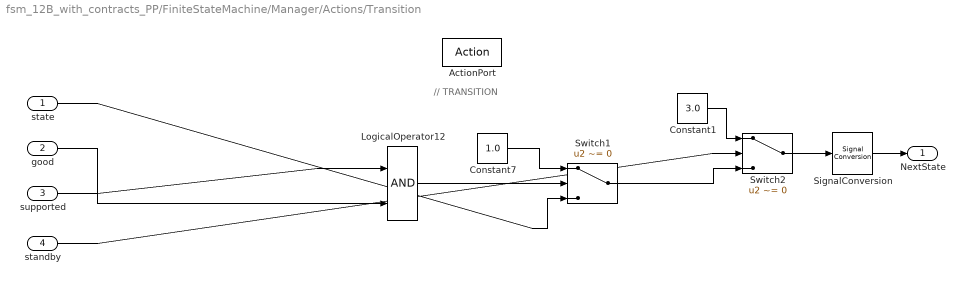
== system fsm_12B_with_contracts_PP/FiniteStateMachine/Manager/Actions/Transition ==
  note: // TRANSITION
  state : Inport
  good : Inport  Port=2
  supported : Inport  Port=3
  standby : Inport  Port=4
  ActionPort : ActionPort
  Constant1 : Constant  Value=3.0
  Constant7 : Constant  Value=1.0
  LogicalOperator12 : Logic  IconShape=distinctive  AllPortsSameDT=off  OutDataTypeStr=boolean
  SignalConversion : SignalConversion  OverrideOpt=off
  Switch1 : Switch  Criteria=u2 ~= 0
  Switch2 : Switch  Criteria=u2 ~= 0
  NextState : Outport  VectorParamsAs1DForOutWhenUnconnected=off
  wires:
  supported/1 -> LogicalOperator12/1
  good/1 -> LogicalOperator12/2
  LogicalOperator12/1 -> Switch1/2
  state/1 -> Switch1/3
  Constant7/1 -> Switch1/1
  standby/1 -> Switch2/2
  Constant1/1 -> Switch2/1
  Switch1/1 -> Switch2/3
  Switch2/1 -> SignalConversion/1
  SignalConversion/1 -> NextState/1

== system fsm_12B_with_contracts_PP/FiniteStateMachine/Manager/Output/Maneuver ==
  note: // Maneuver
  note: PULL
  ActionPort : ActionPort
  Constant10 : Constant  Value=0  OutDataTypeStr=boolean
  Constant11 : Constant  OutDataTypeStr=boolean
  Constant9 : Constant  OutDataTypeStr=boolean
  Mux2 : Mux  Inputs=3
  Output : Outport  VectorParamsAs1DForOutWhenUnconnected=off
  wires:
  Mux2/1 -> Output/1
  Constant10/1 -> Mux2/2
  Constant11/1 -> Mux2/3
  Constant9/1 -> Mux2/1

== system fsm_12B_with_contracts_PP/FiniteStateMachine/Manager/Output/Nominal ==
  note: // Nominal
  note: OPS
  ActionPort : ActionPort
  Constant3 : Constant  OutDataTypeStr=boolean
  Constant4 : Constant  OutDataTypeStr=boolean
  Constant5 : Constant  Value=0  OutDataTypeStr=boolean
  Mux1 : Mux  Inputs=3
  Output : Outport  VectorParamsAs1DForOutWhenUnconnected=off
  wires:
  Constant5/1 -> Mux1/3
  Constant4/1 -> Mux1/2
  Constant3/1 -> Mux1/1
  Mux1/1 -> Output/1

== system fsm_12B_with_contracts_PP/FiniteStateMachine/Manager/Output/Standby ==
  note: PULL
  note: // Standby
  ActionPort : ActionPort
  Constant1 : Constant  Value=0  OutDataTypeStr=boolean
  Constant11 : Constant  Value=0  OutDataTypeStr=boolean
  Constant9 : Constant  OutDataTypeStr=boolean
  Mux2 : Mux  Inputs=3
  Output : Outport  VectorParamsAs1DForOutWhenUnconnected=off
  wires:
  Constant9/1 -> Mux2/1
  Constant11/1 -> Mux2/3
  Constant1/1 -> Mux2/2
  Mux2/1 -> Output/1

== system fsm_12B_with_contracts_PP/FiniteStateMachine/Manager/Output/Transition ==
  note: // TRANSITION
  note: TRANSITION
  ActionPort : ActionPort
  Constant16 : Constant  Value=0  OutDataTypeStr=boolean
  Constant17 : Constant  OutDataTypeStr=boolean
  Constant18 : Constant  Value=0  OutDataTypeStr=boolean
  Mux4 : Mux  Inputs=3
  Output : Outport  VectorParamsAs1DForOutWhenUnconnected=off
  wires:
  Mux4/1 -> Output/1
  Constant17/1 -> Mux4/2
  Constant16/1 -> Mux4/1
  Constant18/1 -> Mux4/3

== system fsm_12B_with_contracts_PP/FiniteStateMachine/Sen/Actions/Fault ==
  note: // Fault
  state : Inport
  request : Inport  Port=2
  limits : Inport  Port=3
  ActionPort : ActionPort
  Constant7 : Constant  Value=1.0
  LogicalOperator12 : Logic  Operator=OR  IconShape=distinctive  AllPortsSameDT=off  OutDataTypeStr=boolean
  LogicalOperator2 : Logic  Operator=NOT  IconShape=distinctive  AllPortsSameDT=off  OutDataTypeStr=boolean
  LogicalOperator3 : Logic  Operator=NOT  IconShape=distinctive  AllPortsSameDT=off  OutDataTypeStr=boolean
  SignalConversion : SignalConversion  OverrideOpt=off
  Switch1 : Switch  Criteria=u2 ~= 0
  NextState : Outport  VectorParamsAs1DForOutWhenUnconnected=off
  wires:
  request/1 -> LogicalOperator2/1
  LogicalOperator12/1 -> Switch1/2
  state/1 -> Switch1/3
  Constant7/1 -> Switch1/1
  Switch1/1 -> SignalConversion/1
  SignalConversion/1 -> NextState/1
  LogicalOperator2/1 -> LogicalOperator12/1
  limits/1 -> LogicalOperator3/1
  LogicalOperator3/1 -> LogicalOperator12/2

== system fsm_12B_with_contracts_PP/FiniteStateMachine/Sen/Actions/Nominal ==
  note: // NOMINAL
  state : Inport
  request : Inport  Port=2
  limits : Inport  Port=3
  ActionPort : ActionPort
  Constant1 : Constant  Value=2.0
  Constant7 : Constant  Value=1.0
  LogicalOperator12 : Logic  Operator=NOT  IconShape=distinctive  AllPortsSameDT=off  OutDataTypeStr=boolean
  SignalConversion : SignalConversion  OverrideOpt=off
  Switch1 : Switch  Criteria=u2 ~= 0
  Switch2 : Switch  Criteria=u2 ~= 0
  NextState : Outport  VectorParamsAs1DForOutWhenUnconnected=off
  wires:
  request/1 -> LogicalOperator12/1
  LogicalOperator12/1 -> Switch1/2
  state/1 -> Switch1/3
  Constant7/1 -> Switch1/1
  limits/1 -> Switch2/2
  Constant1/1 -> Switch2/1
  Switch1/1 -> Switch2/3
  Switch2/1 -> SignalConversion/1
  SignalConversion/1 -> NextState/1

== system fsm_12B_with_contracts_PP/FiniteStateMachine/Sen/Actions/Transition ==
  note: // Transition
  state : Inport
  request : Inport  Port=2
  mode : Inport  Port=3
  ActionPort : ActionPort
  Constant7 : Constant  Value=0.0
  LogicalOperator12 : Logic  IconShape=distinctive  AllPortsSameDT=off  OutDataTypeStr=boolean
  SignalConversion : SignalConversion  OverrideOpt=off
  Switch1 : Switch  Criteria=u2 ~= 0
  NextState : Outport  VectorParamsAs1DForOutWhenUnconnected=off
  wires:
  SignalConversion/1 -> NextState/1
  Switch1/1 -> SignalConversion/1
  Constant7/1 -> Switch1/1
  state/1 -> Switch1/3
  LogicalOperator12/1 -> Switch1/2
  request/1 -> LogicalOperator12/1
  mode/1 -> LogicalOperator12/2

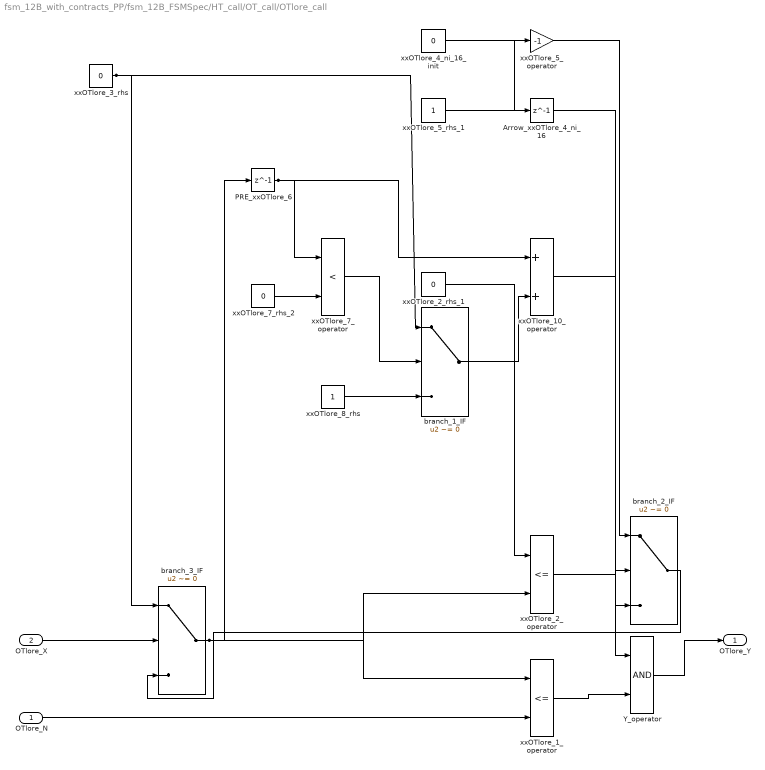
== system fsm_12B_with_contracts_PP/fsm_12B_FSMSpec/HT_call/OT_call/OTlore_call ==
  OTlore_N : Inport
  OTlore_X : Inport  Port=2  OutDataTypeStr=boolean
  Arrow_xxOTlore_4_ni_16 : Delay  DelayLength=1  InitialCondition=1
  PRE_xxOTlore_6 : Delay  DelayLength=1  InitialCondition=0
  Y_operator : Logic  AllPortsSameDT=off  OutDataTypeStr=boolean
  branch_1_IF : Switch  Criteria=u2 ~= 0
  branch_2_IF : Switch  Criteria=u2 ~= 0
  branch_3_IF : Switch  Criteria=u2 ~= 0
  xxOTlore_10_operator : Sum  OutDataTypeStr=int32
  xxOTlore_1_operator : RelationalOperator  Operator=<=  OutDataTypeStr=boolean  RndMeth=Simplest
  xxOTlore_2_operator : RelationalOperator  Operator=<=  OutDataTypeStr=boolean  RndMeth=Simplest
  xxOTlore_2_rhs_1 : Constant  Value=0  OutDataTypeStr=int32
  xxOTlore_3_rhs : Constant  Value=0  OutDataTypeStr=Inherit: Inherit via back propagation
  xxOTlore_4_ni_16_init : Constant  Value=0  OutDataTypeStr=boolean
  xxOTlore_5_operator : Gain  Gain=-1  OutDataTypeStr=int32
  xxOTlore_5_rhs_1 : Constant  OutDataTypeStr=int32
  xxOTlore_7_operator : RelationalOperator  Operator=<  OutDataTypeStr=boolean  RndMeth=Simplest
  xxOTlore_7_rhs_2 : Constant  Value=0  OutDataTypeStr=int32
  xxOTlore_8_rhs : Constant  OutDataTypeStr=Inherit: Inherit via back propagation
  OTlore_Y : Outport
  wires:
  Y_operator/1 -> OTlore_Y/1
  xxOTlore_7_rhs_2/1 -> xxOTlore_7_operator/2
  xxOTlore_5_rhs_1/1 -> xxOTlore_5_operator/1
  xxOTlore_2_rhs_1/1 -> xxOTlore_2_operator/1
  OTlore_N/1 -> xxOTlore_1_operator/2
  branch_1_IF/1 -> xxOTlore_10_operator/2
  branch_2_IF/1 -> branch_3_IF/3
  OTlore_X/1 -> branch_3_IF/2
  xxOTlore_10_operator/1 -> branch_2_IF/3
  Arrow_xxOTlore_4_ni_16/1 -> branch_2_IF/2
  xxOTlore_5_operator/1 -> branch_2_IF/1
  xxOTlore_8_rhs/1 -> branch_1_IF/3
  xxOTlore_7_operator/1 -> branch_1_IF/2
  xxOTlore_1_operator/1 -> Y_operator/2
  xxOTlore_2_operator/1 -> Y_operator/1
  xxOTlore_4_ni_16_init/1 -> Arrow_xxOTlore_4_ni_16/1
  xxOTlore_3_rhs/1 -> branch_3_IF/1, branch_1_IF/1
  PRE_xxOTlore_6/1 -> xxOTlore_7_operator/1, xxOTlore_10_operator/1
  branch_3_IF/1 -> xxOTlore_2_operator/2, xxOTlore_1_operator/1, PRE_xxOTlore_6/1

== system fsm_12B_with_contracts_PP/fsm_12B_FSMSpec/HT_call/OT_call/delay_call ==
  delay_X : Inport  OutDataTypeStr=boolean
  delay_R : Inport  Port=2
  delay_Y : Outport
  wires:
  delay_X/1 -> delay_Y/1
  delay_R/1 -> [delay_R]

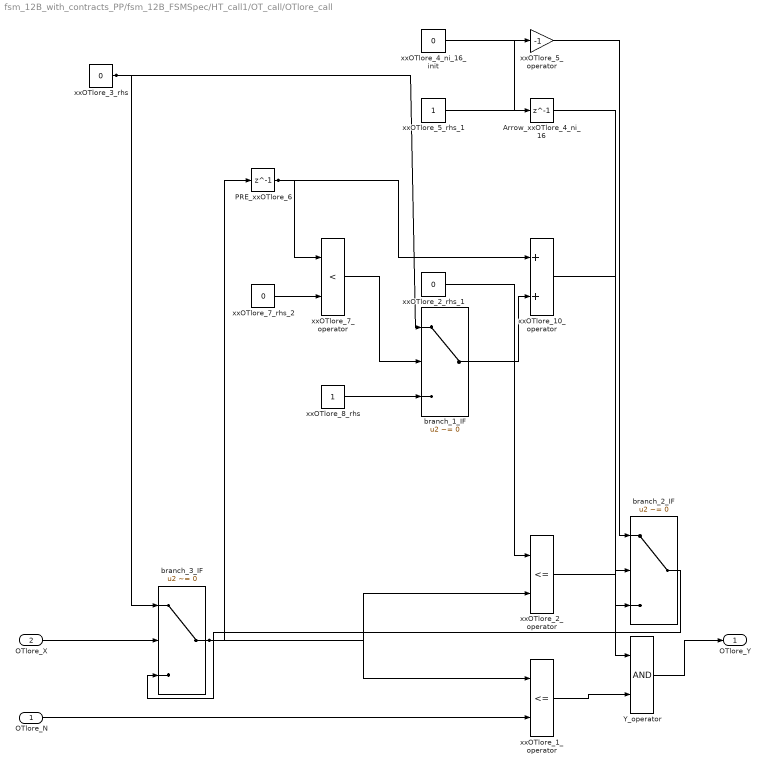
== system fsm_12B_with_contracts_PP/fsm_12B_FSMSpec/HT_call1/OT_call/OTlore_call ==
  OTlore_N : Inport
  OTlore_X : Inport  Port=2  OutDataTypeStr=boolean
  Arrow_xxOTlore_4_ni_16 : Delay  DelayLength=1  InitialCondition=1
  PRE_xxOTlore_6 : Delay  DelayLength=1  InitialCondition=0
  Y_operator : Logic  AllPortsSameDT=off  OutDataTypeStr=boolean
  branch_1_IF : Switch  Criteria=u2 ~= 0
  branch_2_IF : Switch  Criteria=u2 ~= 0
  branch_3_IF : Switch  Criteria=u2 ~= 0
  xxOTlore_10_operator : Sum  OutDataTypeStr=int32
  xxOTlore_1_operator : RelationalOperator  Operator=<=  OutDataTypeStr=boolean  RndMeth=Simplest
  xxOTlore_2_operator : RelationalOperator  Operator=<=  OutDataTypeStr=boolean  RndMeth=Simplest
  xxOTlore_2_rhs_1 : Constant  Value=0  OutDataTypeStr=int32
  xxOTlore_3_rhs : Constant  Value=0  OutDataTypeStr=Inherit: Inherit via back propagation
  xxOTlore_4_ni_16_init : Constant  Value=0  OutDataTypeStr=boolean
  xxOTlore_5_operator : Gain  Gain=-1  OutDataTypeStr=int32
  xxOTlore_5_rhs_1 : Constant  OutDataTypeStr=int32
  xxOTlore_7_operator : RelationalOperator  Operator=<  OutDataTypeStr=boolean  RndMeth=Simplest
  xxOTlore_7_rhs_2 : Constant  Value=0  OutDataTypeStr=int32
  xxOTlore_8_rhs : Constant  OutDataTypeStr=Inherit: Inherit via back propagation
  OTlore_Y : Outport
  wires:
  Y_operator/1 -> OTlore_Y/1
  xxOTlore_7_rhs_2/1 -> xxOTlore_7_operator/2
  xxOTlore_5_rhs_1/1 -> xxOTlore_5_operator/1
  xxOTlore_2_rhs_1/1 -> xxOTlore_2_operator/1
  OTlore_N/1 -> xxOTlore_1_operator/2
  branch_1_IF/1 -> xxOTlore_10_operator/2
  branch_2_IF/1 -> branch_3_IF/3
  OTlore_X/1 -> branch_3_IF/2
  xxOTlore_10_operator/1 -> branch_2_IF/3
  Arrow_xxOTlore_4_ni_16/1 -> branch_2_IF/2
  xxOTlore_5_operator/1 -> branch_2_IF/1
  xxOTlore_8_rhs/1 -> branch_1_IF/3
  xxOTlore_7_operator/1 -> branch_1_IF/2
  xxOTlore_1_operator/1 -> Y_operator/2
  xxOTlore_2_operator/1 -> Y_operator/1
  xxOTlore_4_ni_16_init/1 -> Arrow_xxOTlore_4_ni_16/1
  xxOTlore_3_rhs/1 -> branch_3_IF/1, branch_1_IF/1
  PRE_xxOTlore_6/1 -> xxOTlore_7_operator/1, xxOTlore_10_operator/1
  branch_3_IF/1 -> xxOTlore_2_operator/2, xxOTlore_1_operator/1, PRE_xxOTlore_6/1

== system fsm_12B_with_contracts_PP/fsm_12B_FSMSpec/HT_call1/OT_call/delay_call ==
  delay_X : Inport  OutDataTypeStr=boolean
  delay_R : Inport  Port=2
  delay_Y : Outport
  wires:
  delay_X/1 -> delay_Y/1
  delay_R/1 -> [delay_R]
